simulink model "hw4"  (R2019b)
settings: Solver=VariableStepAuto  StartTime=0.0  StopTime=10  RelTol=1e-3
libraries: simulink x2
settings Model: Creator=scjcb  LastModifiedBy=scjcb

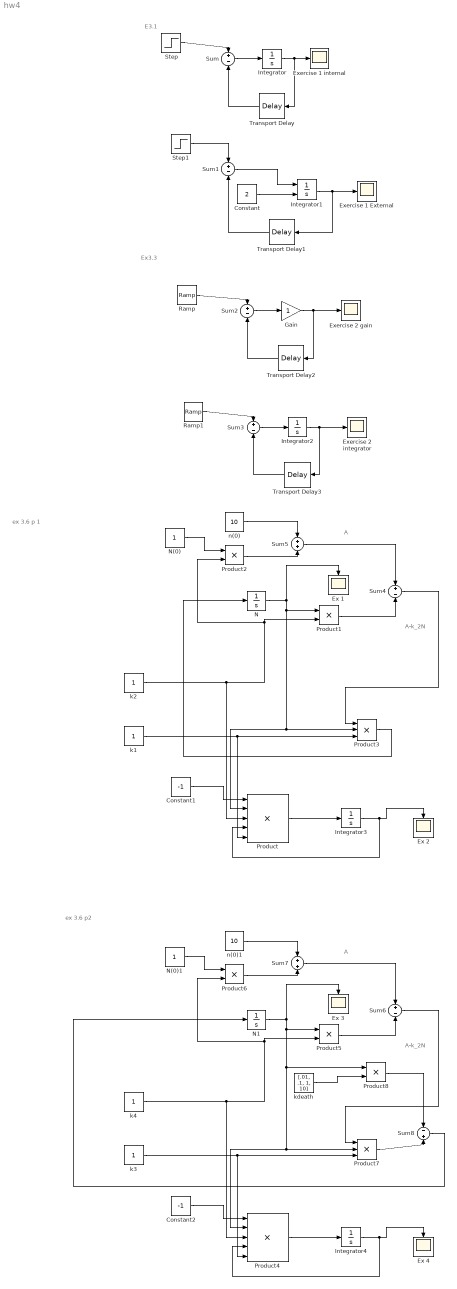
== system hw4 ==
  note: ex 3.6 p2
  note: ex 3.6 p 1
  note: A-k_2N
  note: A
  note: Ex3.3
  note: E3.1
  note: A-k_2N
  note: A
  Constant : Constant  Value=2
  Constant1 : Constant  Value=-1
  Constant2 : Constant  Value=-1
  Ex {1..4} (4 alike) : Scope
  Exercise 1 External : Scope
  Exercise 1 internal : Scope
  Exercise 2 gain : Scope
  Exercise 2 integrator : Scope
  Gain : Gain
  Integrator : Integrator  InitialCondition=2
  Integrator1 : Integrator  InitialConditionSource=external
  Integrator2 : Integrator  InitialCondition=2
  Integrator3 : Integrator  InitialCondition=1
  Integrator4 : Integrator  InitialCondition=1
  N : Integrator  InitialCondition=1
  N(0) : Constant
  N(0)1 : Constant
  N1 : Integrator  InitialCondition=1
  Product : Product  Inputs=*****
  Product1 : Product  Inputs=**
  Product2 : Product
  Product3 : Product  Inputs=***
  Product4 : Product  Inputs=*****
  Product5 : Product  Inputs=**
  Product6 : Product
  Product7 : Product  Inputs=***
  Product8 : Product  Inputs=**
  Ramp : simulink/Sources/Ramp  slope=1  start=0  InitialOutput=0
  Ramp1 : simulink/Sources/Ramp  slope=1  start=0  InitialOutput=0
  Step : Step  SampleTime=0
  Step1 : Step  SampleTime=0
  Sum{,1..4,6} (6 alike) : Sum  Inputs=+-
  Sum5 : Sum
  Sum7 : Sum
  Sum8 : Sum  Inputs=-+
  Transport Delay{,1..3} (4 alike) : TransportDelay  DelayTime=[0.5,1,2]
  k{1..4} (4 alike) : Constant
  kdeath : Constant  Value=[.01, .1, 1, 10]
  n(0) : Constant  Value=10
  n(0)1 : Constant  Value=10
  wires:
  Step/1 -> Sum/1
  Sum/1 -> Integrator/1
  Integrator/1 -> Transport Delay/1, Exercise 1 internal/1
  Transport Delay/1 -> Sum/2
  Transport Delay1/1 -> Sum1/2
  Integrator1/1 -> Exercise 1 External/1, Transport Delay1/1
  Step1/1 -> Sum1/1
  Sum1/1 -> Integrator1/1
  Constant/1 -> Integrator1/2
  Transport Delay2/1 -> Sum2/2
  Gain/1 -> Transport Delay2/1, Exercise 2 gain/1
  Ramp/1 -> Sum2/1
  Sum2/1 -> Gain/1
  Ramp1/1 -> Sum3/1
  Integrator2/1 -> Transport Delay3/1, Exercise 2 integrator/1
  Transport Delay3/1 -> Sum3/2
  Sum3/1 -> Integrator2/1
  k2/1 -> Product1/2, Product2/2, Product/3
  N/1 -> Ex 1/1, Product/2, Product3/2, Product1/1
  n(0)/1 -> Sum5/1
  N(0)/1 -> Product2/1
  Product2/1 -> Sum5/2
  Sum5/1 -> Sum4/1
  Product1/1 -> Sum4/2
  Sum4/1 -> Product3/1
  k1/1 -> Product/5, Product3/3
  Product3/1 -> N/1
  Constant1/1 -> Product/1
  Integrator3/1 -> Ex 2/1, Product/4
  Product/1 -> Integrator3/1
  Product7/1 -> Sum8/2
  Sum6/1 -> Product7/1
  Constant2/1 -> Product4/1
  N(0)1/1 -> Product6/1
  k4/1 -> Product5/2, Product6/2, Product4/3
  N1/1 -> Ex 3/1, Product8/1, Product4/2, Product7/2, Product5/1
  Product4/1 -> Integrator4/1
  k3/1 -> Product4/5, Product7/3
  Product6/1 -> Sum7/2
  Sum7/1 -> Sum6/1
  Integrator4/1 -> Ex 4/1, Product4/4
  Product5/1 -> Sum6/2
  n(0)1/1 -> Sum7/1
  Product8/1 -> Sum8/1
  Sum8/1 -> N1/1
  kdeath/1 -> Product8/2
